simulink model "rx_ovs_ofdm"  (R2022b)
settings: Solver=VariableStepAuto  StartTime=0.0  StopTime=8.3e-3  RelTol=1e-3
undefined symbols (not defined in the file or in its folder): Tovs
libraries: simrfV2util1 x5, dspstat3 x5, simrfV2sources1 x2, simrfV2elements x1
settings Model: SimulationMode=accelerator  Creator=hessam  LastModifiedBy=hessam

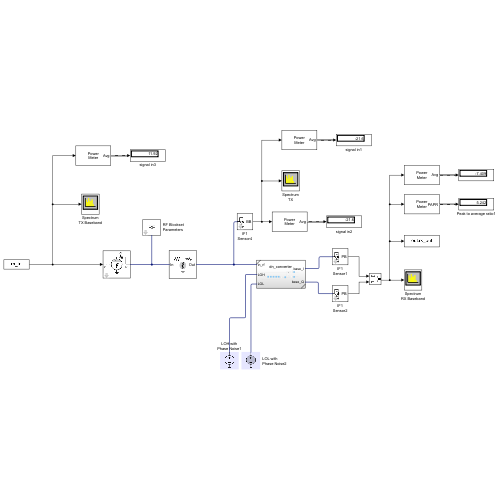
[thumbnail: Simulink's stored preview of the top-level diagram]
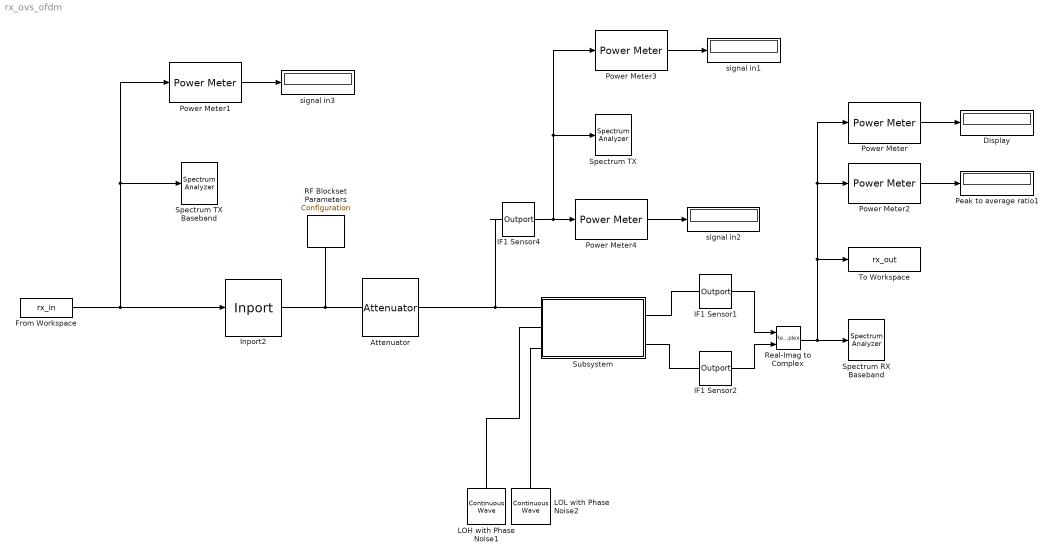
== system rx_ovs_ofdm ==
  Attenuator : simrfV2elements/Attenuator  classname=attenuator  Att=30  Zin=50  Zout=50  AddNoise=on  InternalGrounding=on
  Display : Display
  From Workspace : FromWorkspace  VariableName=rx_in  SampleTime=-1
  IF1 Sensor1 : simrfV2util1/Outport  SensorType=Power  OutputFormat=Real Passband  CarrierFreq=0 Hz  ZL=50  InternalGrounding=on  StepSize=-1 s  AutoStep=off
  IF1 Sensor2 : simrfV2util1/Outport  SensorType=Power  OutputFormat=Real Passband  CarrierFreq=0 Hz  ZL=50  InternalGrounding=on  StepSize=-1 s  AutoStep=off
  IF1 Sensor4 : simrfV2util1/Outport  SensorType=Power  OutputFormat=Complex Baseband  CarrierFreq=carriers.OUT Hz  ZL=50  InternalGrounding=on  StepSize=-1 s  AutoStep=off
  Inport2 : simrfV2util1/Inport  SimulinkInputSignalType=Power  CarrierFreq=carriers.OUT Hz  ZS=50  UseSqWave=off  NumCoeff=10  Bias=0  DutyCyc=50  InternalGrounding=on
  LOH with Phase Noise1 : simrfV2sources1/Continuous Wave  CWSourceType=Ideal voltage  Z0=0  IVoltage=1 V  ICurrent=0 A  MagPower=0 W  QVoltage=0 V  QCurrent=0 A  AnglePower=0  CarrierFreq=carriers.LOH Hz  AddPhaseNoise=off  PhaseNoiseOffset=PhNoOffsets  PhaseNoiseLevel=PhNoLevels  AutoImpulseLength=on  ImpulseLength=1e-10 s  InternalGrounding=on
  LOL with Phase Noise2 : simrfV2sources1/Continuous Wave  CWSourceType=Ideal voltage  Z0=0  IVoltage=1 V  ICurrent=0 A  MagPower=0 W  QVoltage=0 V  QCurrent=0 A  AnglePower=0  CarrierFreq=carriers.LOL Hz  AddPhaseNoise=on  PhaseNoiseOffset=PhNoOffsets  PhaseNoiseLevel=PhNoLevels  AutoImpulseLength=on  ImpulseLength=1e-10 s  InternalGrounding=on
  Peak to average ratio1 : Display
  Power Meter : dspstat3/Power Meter  Measurement=Average power  ReferenceLoad=1  OutputPowerUnits=dBm  WindowLength=1024  OverlapLength=1023  AllowArbitraryInputLength=on  ComputeCCDF=off  PowerRange=50  PowerResolution=0.1  CCDFOutput=Relative power (dB above average power)  ProbabilityVector=[ 10; 1; 0.1; 0.01; 0.001; 0.0001 ]  RelativePowerVector=[ 0; 3; 6; 9; 12 ]  ResetPort=off  SimulateUsing=Code generation
      settings: LibrarySourceBlock=commutil2/Power Meter
  Power Meter1 : dspstat3/Power Meter  Measurement=Average power  ReferenceLoad=1  OutputPowerUnits=dBm  WindowLength=256  OverlapLength=255  AllowArbitraryInputLength=on  ComputeCCDF=off  PowerRange=50  PowerResolution=0.1  CCDFOutput=Relative power (dB above average power)  ProbabilityVector=[ 10; 1; 0.1; 0.01; 0.001; 0.0001 ]  RelativePowerVector=[ 0; 3; 6; 9; 12 ]  ResetPort=off  SimulateUsing=Code generation
      settings: LibrarySourceBlock=commutil2/Power Meter
  Power Meter2 : dspstat3/Power Meter  Measurement=Peak-to-average power ratio  ReferenceLoad=1  OutputPowerUnits=dBm  WindowLength=256  OverlapLength=255  AllowArbitraryInputLength=on  ComputeCCDF=off  PowerRange=50  PowerResolution=0.1  CCDFOutput=Relative power (dB above average power)  ProbabilityVector=[ 10; 1; 0.1; 0.01; 0.001; 0.0001 ]  RelativePowerVector=[ 0; 3; 6; 9; 12 ]  ResetPort=off  SimulateUsing=Code generation
      settings: LibrarySourceBlock=commutil2/Power Meter
  Power Meter3 : dspstat3/Power Meter  Measurement=Average power  ReferenceLoad=1  OutputPowerUnits=dBm  WindowLength=256  OverlapLength=255  AllowArbitraryInputLength=on  ComputeCCDF=off  PowerRange=50  PowerResolution=0.1  CCDFOutput=Relative power (dB above average power)  ProbabilityVector=[ 10; 1; 0.1; 0.01; 0.001; 0.0001 ]  RelativePowerVector=[ 0; 3; 6; 9; 12 ]  ResetPort=off  SimulateUsing=Code generation
      settings: LibrarySourceBlock=commutil2/Power Meter
  Power Meter4 : dspstat3/Power Meter  Measurement=Average power  ReferenceLoad=1  OutputPowerUnits=dBm  WindowLength=256  OverlapLength=255  AllowArbitraryInputLength=on  ComputeCCDF=off  PowerRange=50  PowerResolution=0.1  CCDFOutput=Relative power (dB above average power)  ProbabilityVector=[ 10; 1; 0.1; 0.01; 0.001; 0.0001 ]  RelativePowerVector=[ 0; 3; 6; 9; 12 ]  ResetPort=off  SimulateUsing=Code generation
      settings: LibrarySourceBlock=commutil2/Power Meter
  RF Blockset Parameters : simrfV2util1/Configuration  AutoFreq=on  Tones="[11  66] GHz"  Harmonics="[5  5]"  NormalizeCarrierPower=on  SolverType=Auto  UseCCode=on  StepSize=Tovs s  AddNoise=off  defaultRNG=on  Seed=0  Temperature=293.15 K  SolverDelFlag=0  AbsTol=1e-6  RelTol=1e-3  MaxIter=10  ErrorEstimationType=2-norm over all variables  EnableInterpFilter=off  HiddenFIRfilterControllerParam=on  SmallSignalApprox=off  AllSimFreqs=on  SimFreqs=[] Hz  SimFreqsInternal=[]  SamplesPerFrame=1
  Real-Imag to Complex : RealImagToComplex
  Spectrum RX Baseband : SpectrumAnalyzer
  Spectrum TX : SpectrumAnalyzer
  Spectrum TX Baseband : SpectrumAnalyzer
  Subsystem : Subsystem  ReferencedSubsystem=dn_converter
      settings: PortSchema="{\"entries\":[{\"content\":{\"sides\":[{\"content\":{\"connectorIds\":[\"LConn3\",\"LConn1\",\"LConn2\"]},\"type\":\"ConnectorPlacement.EquallySpacedRectSide\",\"uuid\":\"8336b51e-e5d8-49cc-804f-7bfb99400ab0\"},{\"content\":{\"connectorIds\":[\"LConn4\",\"LConn5\"],\"side\":\"RIGHT\"},\"type\":\"ConnectorPlacement.EquallySpacedRectSide\",\"uuid\":\"6f005c77-3014-47d2-89f9-41814728faba\"},{\"content\":{\"connectorIds\":[],\"side\":\"TOP\"},\"type\":\"ConnectorPlacement.EquallySpacedRectSide\",\"uuid\":\"edcdef5b-1b73-4458-84fc-72d761e40cdf\"}]},\"type\":\"ConnectorPlacement.EquallySpacedConnector\",\"uuid\":\"3f0b5c66-2f3f-40e5-bb1c-488293219f70\"}],\"packageUris\":[\"http://schema.mathworks.com/mf0/Connector/R2020b\"],\"version\":\"1.0\"}"
  To Workspace : ToWorkspace  VariableName=rx_out  SampleTime=-1
  signal in1 : Display
  signal in2 : Display
  signal in3 : Display
  wires:
  IF1 Sensor1/1 -> Real-Imag to Complex/1
  Power Meter/1 -> Display/1
  Real-Imag to Complex/1 -> To Workspace/1, Power Meter2/1, Power Meter/1, Spectrum RX Baseband/1
  Power Meter2/1 -> Peak to average ratio1/1
  IF1 Sensor2/1 -> Real-Imag to Complex/2
  Power Meter3/1 -> signal in1/1
  Power Meter4/1 -> signal in2/1
  IF1 Sensor4/1 -> Spectrum TX/1, Power Meter3/1, Power Meter4/1
  From Workspace/1 -> Inport2/1, Power Meter1/1, Spectrum TX Baseband/1
  Power Meter1/1 -> signal in3/1
  connections:
  Inport2/RConn1 -- RF Blockset Parameters/LConn1 -- Attenuator/LConn1
  Subsystem/LConn3 -- IF1 Sensor4/LConn1 -- Attenuator/RConn1
  LOH with Phase Noise1/LConn1 -- Subsystem/LConn1
  Subsystem/LConn2 -- LOL with Phase Noise2/LConn1
  Subsystem/LConn5 -- IF1 Sensor2/LConn1
  Subsystem/LConn4 -- IF1 Sensor1/LConn1
